simulink model "full_maneuver_single_veh"  (R2020a)
settings: Solver=VariableStepAuto  StartTime=0.0  StopTime=90  FixedStep=0.1  MaxStep=5e-2  RelTol=1e-3
InitFcn:
  | totalVehicles = 5;
  | if exist('vehStatesBus', 'var')==0
  | load vehBuses
  | end
  | if exist('vehErrorsBus', 'var')==0
  | load vehBuses
  | end
libraries: simulink x69, powerlib_meascontrol x6, autolibshared x6, dspsigops x3, eeGeneralControl x2
(part 4 of 6)

== system full_maneuver_single_veh/Fd/Virtual Vehicle Following/Min Velocity Control ==
  ev : Inport
  ea : Inport  Port=2
  realInput : Inport  Port=3
  Abs : Abs
  Compare To Constant : simulink/Logic and Bit Operations/Compare To Constant  relop=<=  const=0.2  OutDataTypeStr=boolean
  Gain : Gain  Gain=velKd
  Scope : Scope  NumInputPorts=4
  Sum1 : Sum  Inputs=|-+
  Sum3 : Sum  Inputs=+++
  Transport Delay : TransportDelay  DelayTime=0.1
  integral term : Subsystem
  velKp : Gain  Gain=velKp
  u : Outport  VectorParamsAs1DForOutWhenUnconnected=off
  wires:
  Gain/1 -> Sum3/3, Scope/3
  ea/1 -> Gain/1
  realInput/1 -> Sum1/1
  Sum3/1 -> u/1, Transport Delay/1, Scope/4
  velKp/1 -> Sum3/2, Scope/2
  ev/1 -> integral term/1(ev), velKp/1
  Sum1/1 -> Abs/1
  Abs/1 -> Compare To Constant/1
  integral term/1(Out1) -> Scope/1, Sum3/1
  Compare To Constant/1 -> integral term/Enable
  Transport Delay/1 -> Sum1/2

== system full_maneuver_single_veh/Fd/Virtual Vehicle Following/Min Velocity Error ==
  ego : Inport
  velRef : Inport  Port=2
  filterReset : Inport  Port=3
  Bus Selector : BusSelector  OutputSignals=Xdot,xddot
  Gain : Gain  Gain=-1
  Gain3 : Gain  Gain=velFilterGain
  Integrator1 : Integrator  ExternalReset=rising  InitialCondition=vx0
  Saturation : Saturate  UpperLimit=maxComfAccel  LowerLimit=minComfAccel
  Sum : Sum  Inputs=+-|
  Sum8 : Sum  Inputs=|+-
  ev : Outport
  ea : Outport  Port=2
  wires:
  Sum8/1 -> Gain3/1
  Gain3/1 -> Saturation/1
  Saturation/1 -> Integrator1/1
  velRef/1 -> Sum8/1
  Integrator1/1 -> Sum/1, Sum8/2
  ego/1 -> Bus Selector/1
  Bus Selector/1 -> Sum/2  "<Xdot>"
  Bus Selector/2 -> Gain/1  "<xddot>"
  Sum/1 -> ev/1
  Gain/1 -> ea/1
  filterReset/1 -> Integrator1/2

== system full_maneuver_single_veh/Fd/Virtual Vehicle Following/Virtual Leader Following ==
  errors : Inport
  errorsDot : Inport  Port=2
  realInput : Inport  Port=3
  leaderChange : Inport  Port=4
  inRange : Inport  Port=5
  Demux : Demux  Outputs=2
  Demux1 : Demux  Outputs=2
  Gain : Gain  Gain=10
  Gain3 : Gain  Gain=Ka
  Gain4 : Gain  Gain=Kdd
  Gain5 : Gain  Gain=10
  Integrator1 : Integrator  ExternalReset=rising  InitialConditionSource=external  InitialCondition=vx0
  Integrator2 : Integrator  ExternalReset=rising
  Kd : Gain  Gain=Kd
  Kp : Gain  Gain=Kp
  Saturation : Saturate  UpperLimit=maxComfAccel  LowerLimit=minAcceleration
  Saturation1 : Saturate  UpperLimit=maxGapError  LowerLimit=-maxGapError*2
  Scope : Scope  NumInputPorts=6
  Sum : Sum  Inputs=+-|
  Sum1 : Sum  Inputs=+++++
  Sum8 : Sum  Inputs=|+-
  Sum9 : Sum  Inputs=|+-
  Transport Delay : TransportDelay  DelayTime=0.1
  integralTerm : Subsystem
  u : Outport  VectorParamsAs1DForOutWhenUnconnected=off
  wires:
  Demux1/2 -> Gain3/1  "evDot"
  Demux1/1 -> Gain4/1  "egDot"
  leaderChange/1 -> integralTerm/3(leaderChange), Integrator2/2
  integralTerm/1(Out1) -> Transport Delay/1
  Sum1/1 -> Sum8/1, Scope/6, Sum/1
  Integrator1/1 -> Sum8/2, u/1
  Gain3/1 -> Sum1/5, Scope/5
  Demux/2 -> Kd/1  "ev"
  Saturation/1 -> Integrator1/1
  Gain4/1 -> Sum1/4, Scope/4
  realInput/1 -> Sum/2, Integrator1/3
  Sum8/1 -> Gain5/1
  Sum/1 -> integralTerm/2(inputDiff)
  Kp/1 -> Sum1/2, Scope/2
  Integrator2/1 -> Sum9/2, Kp/1, integralTerm/1(eh)
  Transport Delay/1 -> Sum1/1, Scope/1
  inRange/1 -> Integrator1/2, integralTerm/Enable
  Gain5/1 -> Saturation/1
  Kd/1 -> Sum1/3, Scope/3
  Demux/1 -> Saturation1/1
  Gain/1 -> Integrator2/1
  Sum9/1 -> Gain/1
  Saturation1/1 -> Sum9/1
  errors/1 -> Demux/1
  errorsDot/1 -> Demux1/1

== system full_maneuver_single_veh/Fd/Virtual Vehicle Following/switch min vel ==
  errors : Inport
  errorsDot : Inport  Port=2
  gap : Inport  Port=3
  h : Inport  Port=4
  d0 : Inport  Port=5
  vRef : Inport  Port=6
  Demux1 : Demux  Outputs=2
  Gain1 : Gain
  MATLAB Function : MATLAB Function  TreatAsAtomicUnit=on
  Relay1 : Relay  OnSwitchValue=1  OffSwitchValue=-1
  Scope : Scope  NumInputPorts=2
  Scope1 : Scope  NumInputPorts=2
  Selector : Selector  InputPortWidth=2  IndexOptions=Index vector (dialog)  Indices=[2]  OutputSizes=1
  Sum2 : Sum  Inputs=-+
  inRange : Outport  VectorParamsAs1DForOutWhenUnconnected=off
  wires:
  d0/1 -> MATLAB Function/2(d0)
  vRef/1 -> MATLAB Function/3(vRef)
  h/1 -> Gain1/1
  errors/1 -> Selector/1
  gap/1 -> Scope/1, Sum2/1
  Sum2/1 -> Scope1/1, Relay1/1
  Selector/1 -> MATLAB Function/4(ev)
  Relay1/1 -> inRange/1, Scope1/2
  Gain1/1 -> MATLAB Function/1(h)
  MATLAB Function/1(maxGap) -> Scope/2, Sum2/2
  errorsDot/1 -> Demux1/1
  Demux1/1 -> MATLAB Function/5(ehDot)
  Demux1/2 -> MATLAB Function/6(ea)

== system full_maneuver_single_veh/Fd_bkp/Find Leader/Subsystem ==
  ego : Inport
  all : Inport  Port=2
  Enable : EnablePort
  MATLAB Function : MATLAB Function  TreatAsAtomicUnit=on
  idx : Outport  InitialOutput=1  VectorParamsAs1DForOutWhenUnconnected=off
  wires:
  all/1 -> MATLAB Function/2(allVehicles)
  MATLAB Function/1(leaderIdx) -> idx/1
  ego/1 -> MATLAB Function/1(ego)

== system full_maneuver_single_veh/Fd_bkp/Find Leader/farAwayVeh ==
  ego : Inport  OutDataTypeStr=Bus: vehStatesBus
  Bus Assignment : BusAssignment  AssignedSignals=X
  Bus Selector : BusSelector  OutputSignals=X
  Constant : Constant  Value=1000
  Sum : Sum  Inputs=|++
  Out1 : Outport  OutDataTypeStr=Bus: vehStatesBus  VectorParamsAs1DForOutWhenUnconnected=off
  wires:
  Sum/1 -> Bus Assignment/2  "X"
  Bus Selector/1 -> Sum/1  "<X>"
  Bus Assignment/1 -> Out1/1
  Constant/1 -> Sum/2
  ego/1 -> Bus Selector/1, Bus Assignment/1

== system full_maneuver_single_veh/Fd_bkp/Lateral Control/Full State Observer ==
  note: xhat
  note: yhat
  measuredOutputs : Inport
  delta : Inport  Port=2
  Add1 : Sum  Inputs=|-+
  Gain : Gain  Gain=B  Multiplication=Matrix(K*u)
  Gain1 : Gain  Gain=C  Multiplication=Matrix(K*u)
  Gain2 : Gain  Gain=L  Multiplication=Matrix(K*u)
  Gain3 : Gain  Gain=A  Multiplication=Matrix(K*u)
  Integrator : Integrator  InitialCondition=[y0; 0; 0; 0]
  Signal Specification : SignalSpecification  Dimensions=[size(C,1) 1]
  Sum : Sum  Inputs=+++
  xhat : Outport  VectorParamsAs1DForOutWhenUnconnected=off
  wires:
  Add1/1 -> Signal Specification/1
  Integrator/1 -> xhat/1, Gain3/1, Gain1/1
  Gain1/1 -> Add1/1
  Sum/1 -> Integrator/1
  measuredOutputs/1 -> Add1/2
  delta/1 -> Gain/1
  Gain/1 -> Sum/3
  Gain3/1 -> Sum/2
  Signal Specification/1 -> Gain2/1
  Gain2/1 -> Sum/1

== system full_maneuver_single_veh/Fd_bkp/Maneuver State/Triggered Subsystem ==
  Trigger : TriggerPort  VariantControl=Variant
  Constant : Constant  OutDataTypeStr=fixdt(1,16,0)
  Out1 : Outport  InitialOutput=0  VectorParamsAs1DForOutWhenUnconnected=off
  wires:
  Constant/1 -> Out1/1

== system full_maneuver_single_veh/Fd_bkp/Maneuver State/Triggered Subsystem1 ==
  Trigger : TriggerPort  VariantControl=Variant
  Constant : Constant  Value=true  OutDataTypeStr=boolean
  Out1 : Outport  OutDataTypeStr=boolean  InitialOutput=0  VectorParamsAs1DForOutWhenUnconnected=off
  wires:
  Constant/1 -> Out1/1

== system full_maneuver_single_veh/Fd_bkp/Maneuver State/safeErrors ==
  errors : Inport
  AND : Logic  Inputs=1  IconShape=distinctive  AllPortsSameDT=off  OutDataTypeStr=boolean
  Compare To Constant4 : simulink/Logic and Bit Operations/Compare To Constant  relop=>=  const=-0.1  OutDataTypeStr=boolean
  Memory : Memory
  Triggered Subsystem1 : Subsystem  TreatAsAtomicUnit=on
  safetyFlag : Outport  VectorParamsAs1DForOutWhenUnconnected=off
  wires:
  Memory/1 -> safetyFlag/1
  Triggered Subsystem1/1(Out1) -> Memory/1
  errors/1 -> Compare To Constant4/1
  AND/1 -> Triggered Subsystem1/Trigger
  Compare To Constant4/1 -> AND/1

== system full_maneuver_single_veh/Fd_bkp/Maneuver State/safeErrors1 ==
  errors : Inport
  AND : Logic  Inputs=1  IconShape=distinctive  AllPortsSameDT=off  OutDataTypeStr=boolean
  Compare To Constant4 : simulink/Logic and Bit Operations/Compare To Constant  relop=>=  const=-0.1  OutDataTypeStr=boolean
  safetyFlag : Outport  VectorParamsAs1DForOutWhenUnconnected=off
  wires:
  AND/1 -> safetyFlag/1
  errors/1 -> Compare To Constant4/1
  Compare To Constant4/1 -> AND/1

== system full_maneuver_single_veh/Fd_bkp/Maneuver State/safeErrors2 ==
  errors : Inport
  AND : Logic  Inputs=1  IconShape=distinctive  AllPortsSameDT=off  OutDataTypeStr=boolean
  Compare To Constant4 : simulink/Logic and Bit Operations/Compare To Constant  relop=>=  const=-0.1  OutDataTypeStr=boolean
  safetyFlag : Outport  VectorParamsAs1DForOutWhenUnconnected=off
  wires:
  errors/1 -> Compare To Constant4/1
  AND/1 -> safetyFlag/1
  Compare To Constant4/1 -> AND/1

== system full_maneuver_single_veh/Fd_bkp/Maneuver State/steadyState ==
  u : Inport
  AND : Logic  Inputs=1  IconShape=distinctive  AllPortsSameDT=off  OutDataTypeStr=boolean
  Abs2 : Abs
  Compare To Constant2 : simulink/Logic and Bit Operations/Compare To Constant  relop=<=  const=0.2  OutDataTypeStr=boolean
  Mux : Mux  Inputs=2
  Transport Delay2 : TransportDelay
  ssFlag : Outport  VectorParamsAs1DForOutWhenUnconnected=off
  wires:
  Mux/1 -> Abs2/1
  AND/1 -> ssFlag/1
  Transport Delay2/1 -> Mux/1
  Abs2/1 -> Compare To Constant2/1
  u/1 -> Mux/2, Transport Delay2/1
  Compare To Constant2/1 -> AND/1

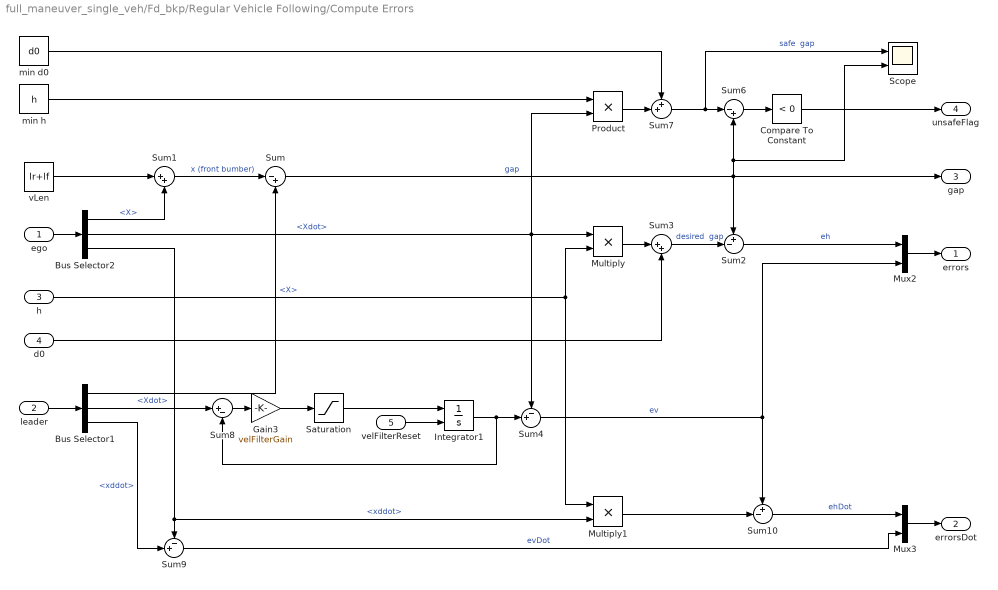
== system full_maneuver_single_veh/Fd_bkp/Regular Vehicle Following/Compute Errors ==
  ego : Inport
  leader : Inport  Port=2
  h : Inport  Port=3
  d0 : Inport  Port=4
  velFilterReset : Inport  Port=5
  Bus Selector1 : BusSelector  OutputSignals=X,Xdot,xddot
  Bus Selector2 : BusSelector  OutputSignals=X,Xdot,xddot
  Compare To Constant : simulink/Logic and Bit Operations/Compare To Constant  relop=<  const=0  OutDataTypeStr=boolean
  Gain3 : Gain  Gain=velFilterGain
  Integrator1 : Integrator  ExternalReset=rising  InitialCondition=vx0
  Multiply : Product
  Multiply1 : Product
  Mux2 : Mux  Inputs=2
  Mux3 : Mux  Inputs=2
  Product : Product
  Saturation : Saturate  UpperLimit=maxAcceleration  LowerLimit=minAcceleration
  Scope : Scope  NumInputPorts=2
  Sum : Sum  Inputs=|-+
  Sum1 : Sum  Inputs=|++
  Sum10 : Sum  Inputs=+-|
  Sum2 : Sum  Inputs=+-|
  Sum3 : Sum  Inputs=|++
  Sum4 : Sum  Inputs=-+|
  Sum6 : Sum  Inputs=|-+
  Sum7 : Sum  Inputs=++|
  Sum8 : Sum  Inputs=|+-
  Sum9 : Sum  Inputs=-+|
  min d0 : Constant  Value=d0
  min h : Constant  Value=h
  vLen : Constant  Value=lr+lf
  errors : Outport  VectorParamsAs1DForOutWhenUnconnected=off
  errorsDot : Outport  Port=2
  "gap " : Outport  Port=3  VectorParamsAs1DForOutWhenUnconnected=off
  unsafeFlag : Outport  Port=4  VectorParamsAs1DForOutWhenUnconnected=off
  wires:
  Mux2/1 -> errors/1
  velFilterReset/1 -> Integrator1/2
  Sum6/1 -> Compare To Constant/1
  Sum7/1 -> Sum6/1, Scope/1  "safe  gap"
  min h/1 -> Product/1
  Compare To Constant/1 -> unsafeFlag/1
  Sum2/1 -> Mux2/1  "eh"
  Bus Selector1/1 -> Sum/2  "<X>"
  Product/1 -> Sum7/2
  Sum3/1 -> Sum2/2  "desired  gap"
  Sum1/1 -> Sum/1  "x (front bumber)"
  Bus Selector2/2 -> Sum4/1, Multiply/1, Product/2  "<Xdot>"
  d0/1 -> Sum3/2
  vLen/1 -> Sum1/1
  min d0/1 -> Sum7/1
  Multiply/1 -> Sum3/1
  Sum/1 -> Sum2/1, "gap "/1, Sum6/2, Scope/2  "gap"
  Bus Selector2/1 -> Sum1/2  "<X>"
  h/1 -> Multiply/2, Multiply1/1
  Bus Selector1/2 -> Sum8/1  "<Xdot>"
  Sum4/1 -> Mux2/2, Sum10/1  "ev"
  Gain3/1 -> Saturation/1
  Saturation/1 -> Integrator1/1
  Integrator1/1 -> Sum4/2, Sum8/2
  Sum8/1 -> Gain3/1
  Bus Selector1/3 -> Sum9/2  "<xddot>"
  Bus Selector2/3 -> Sum9/1, Multiply1/2  "<xddot>"
  Multiply1/1 -> Sum10/2
  Sum10/1 -> Mux3/1  "ehDot"
  Sum9/1 -> Mux3/2  "evDot"
  Mux3/1 -> errorsDot/1
  ego/1 -> Bus Selector2/1
  leader/1 -> Bus Selector1/1

== system full_maneuver_single_veh/Fd_bkp/Regular Vehicle Following/Define Desired Distance ==
  extraSpaceFlag : Inport
  Constant : Constant  Value=h
  Constant1 : Constant  Value=d0
  Constant2 : Constant  Value=hLC
  Constant3 : Constant  Value=d0LC
  Demux : Demux  Outputs=2
  Integrator : Integrator  InitialCondition=[h d0]
  Mux : Mux  Inputs=2
  Mux1 : Mux  Inputs=2
  Saturation1 : Saturate  UpperLimit=hFilterSaturation  LowerLimit=-hFilterSaturation
  Sum5 : Sum  Inputs=|+-
  Switch : Switch  Criteria=u2 > Threshold
  hFilterGain : Gain  Gain=hFilterGain
  h : Outport
  d0 : Outport  Port=2
  wires:
  Mux/1 -> Switch/3
  Constant/1 -> Mux/1
  hFilterGain/1 -> Saturation1/1
  Constant2/1 -> Mux1/1
  Sum5/1 -> hFilterGain/1
  Mux1/1 -> Switch/1
  Switch/1 -> Sum5/1
  Constant3/1 -> Mux1/2
  Constant1/1 -> Mux/2
  extraSpaceFlag/1 -> Switch/2
  Saturation1/1 -> Integrator/1
  Integrator/1 -> Demux/1, Sum5/2
  Demux/1 -> h/1
  Demux/2 -> d0/1

== system full_maneuver_single_veh/Fd_bkp/Regular Vehicle Following/Veh Following ==
  errors : Inport
  errorsDot : Inport  Port=2
  realInput : Inport  Port=3
  leaderChange : Inport  Port=4
  inRange : Inport  Port=5
  Demux : Demux  Outputs=2
  Demux1 : Demux  Outputs=2
  Gain : Gain  Gain=Ka
  Gain1 : Gain  Gain=Kdd
  Kd : Gain  Gain=Kd
  Kp : Gain  Gain=Kp
  Saturation1 : Saturate  UpperLimit=maxHeadwayError  LowerLimit=minHeadwayError
  Scope : Scope  NumInputPorts=6
  Sum : Sum  Inputs=|-+
  Sum1 : Sum  Inputs=+++
  Sum2 : Sum  Inputs=|++
  Sum3 : Sum  Inputs=|++
  Transport Delay : TransportDelay  DelayTime=0.1
  integralTerm : Subsystem
  u : Outport  VectorParamsAs1DForOutWhenUnconnected=off
  wires:
  inRange/1 -> integralTerm/Enable
  errors/1 -> Demux/1
  Saturation1/1 -> integralTerm/1(eh), Kp/1
  Demux/2 -> Kd/1  "ev"
  Kp/1 -> Sum1/2, Scope/2
  Kd/1 -> Scope/3, Sum1/3
  Demux/1 -> Saturation1/1  "eh"
  leaderChange/1 -> integralTerm/2(leaderChange)
  Transport Delay/1 -> Sum1/1, Scope/1
  Sum1/1 -> Sum3/1
  realInput/1 -> Sum/1
  Sum/1 -> integralTerm/3(inputDiff)
  integralTerm/1(Out1) -> Transport Delay/1
  Gain1/1 -> Scope/4, Sum2/1
  Gain/1 -> Scope/5, Sum2/2
  Sum3/1 -> Scope/6, Sum/2, u/1
  Sum2/1 -> Sum3/2
  errorsDot/1 -> Demux1/1
  Demux1/1 -> Gain1/1  "ehDot"
  Demux1/2 -> Gain/1  "evDot"

== system full_maneuver_single_veh/Fd_bkp/Regular Vehicle Following/Velocity Control ==
  ev : Inport
  ea : Inport  Port=2
  realInput : Inport  Port=3
  Abs : Abs
  Compare To Constant : simulink/Logic and Bit Operations/Compare To Constant  relop=<=  const=0.5  OutDataTypeStr=boolean
  Gain : Gain  Gain=velKd
  Scope : Scope  NumInputPorts=4
  Sum1 : Sum  Inputs=|-+
  Sum3 : Sum  Inputs=+++
  Transport Delay : TransportDelay  DelayTime=0.1
  integral term : Subsystem
  velKp : Gain  Gain=velKp
  u : Outport  VectorParamsAs1DForOutWhenUnconnected=off
  wires:
  Gain/1 -> Sum3/3, Scope/3
  ea/1 -> Gain/1
  realInput/1 -> Sum1/1
  Sum3/1 -> u/1, Transport Delay/1, Scope/4
  velKp/1 -> Sum3/2, Scope/2
  ev/1 -> integral term/1(ev), velKp/1
  Sum1/1 -> Abs/1
  Abs/1 -> Compare To Constant/1
  integral term/1(Out1) -> Scope/1, Sum3/1
  Compare To Constant/1 -> integral term/Enable
  Transport Delay/1 -> Sum1/2

== system full_maneuver_single_veh/Fd_bkp/Regular Vehicle Following/switch free flow ==
  errors : Inport
  errorsDot : Inport  Port=2
  gap : Inport  Port=3
  h : Inport  Port=4
  d0 : Inport  Port=5
  vRef : Inport  Port=6
  Demux1 : Demux  Outputs=2
  Gain1 : Gain
  MATLAB Function : MATLAB Function  TreatAsAtomicUnit=on
  Relay : Relay  OnSwitchValue=1  OffSwitchValue=-1
  Scope : Scope  NumInputPorts=2
  Selector : Selector  InputPortWidth=2  IndexOptions=Index vector (dialog)  Indices=[2]  OutputSizes=1
  Sum2 : Sum  Inputs=-+
  inRange : Outport  VectorParamsAs1DForOutWhenUnconnected=off
  wires:
  d0/1 -> MATLAB Function/2(d0)
  vRef/1 -> MATLAB Function/3(vRef)
  h/1 -> Gain1/1
  errors/1 -> Selector/1
  gap/1 -> Scope/1, Sum2/1
  Sum2/1 -> Relay/1
  Selector/1 -> MATLAB Function/4(ev)
  Relay/1 -> inRange/1
  Gain1/1 -> MATLAB Function/1(h)
  MATLAB Function/1(maxGap) -> Scope/2, Sum2/2
  errorsDot/1 -> Demux1/1
  Demux1/1 -> MATLAB Function/5(ehDot)
  Demux1/2 -> MATLAB Function/6(ea)

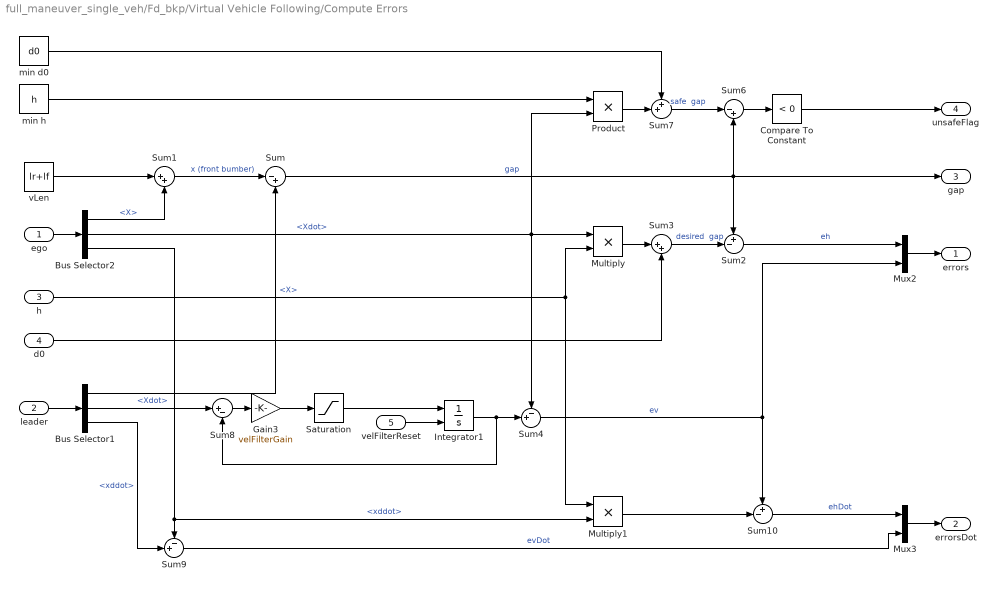
== system full_maneuver_single_veh/Fd_bkp/Virtual Vehicle Following/Compute Errors ==
  ego : Inport
  leader : Inport  Port=2
  h : Inport  Port=3
  d0 : Inport  Port=4
  velFilterReset : Inport  Port=5
  Bus Selector1 : BusSelector  OutputSignals=X,Xdot,xddot
  Bus Selector2 : BusSelector  OutputSignals=X,Xdot,xddot
  Compare To Constant : simulink/Logic and Bit Operations/Compare To Constant  relop=<  const=0  OutDataTypeStr=boolean
  Gain3 : Gain  Gain=velFilterGain
  Integrator1 : Integrator  ExternalReset=rising  InitialCondition=vx0
  Multiply : Product
  Multiply1 : Product
  Mux2 : Mux  Inputs=2
  Mux3 : Mux  Inputs=2
  Product : Product
  Saturation : Saturate  UpperLimit=maxAcceleration  LowerLimit=minAcceleration
  Sum : Sum  Inputs=|-+
  Sum1 : Sum  Inputs=|++
  Sum10 : Sum  Inputs=+-|
  Sum2 : Sum  Inputs=+-|
  Sum3 : Sum  Inputs=|++
  Sum4 : Sum  Inputs=-+|
  Sum6 : Sum  Inputs=|-+
  Sum7 : Sum  Inputs=++|
  Sum8 : Sum  Inputs=|+-
  Sum9 : Sum  Inputs=-+|
  min d0 : Constant  Value=d0
  min h : Constant  Value=h
  vLen : Constant  Value=lr+lf
  errors : Outport  VectorParamsAs1DForOutWhenUnconnected=off
  errorsDot : Outport  Port=2
  "gap " : Outport  Port=3  VectorParamsAs1DForOutWhenUnconnected=off
  unsafeFlag : Outport  Port=4  VectorParamsAs1DForOutWhenUnconnected=off
  wires:
  Mux2/1 -> errors/1
  velFilterReset/1 -> Integrator1/2
  Sum6/1 -> Compare To Constant/1
  Sum7/1 -> Sum6/1  "safe  gap"
  min h/1 -> Product/1
  Compare To Constant/1 -> unsafeFlag/1
  Sum2/1 -> Mux2/1  "eh"
  Bus Selector1/1 -> Sum/2  "<X>"
  Product/1 -> Sum7/2
  Sum3/1 -> Sum2/2  "desired  gap"
  Sum1/1 -> Sum/1  "x (front bumber)"
  Bus Selector2/2 -> Sum4/1, Multiply/1, Product/2  "<Xdot>"
  d0/1 -> Sum3/2
  vLen/1 -> Sum1/1
  min d0/1 -> Sum7/1
  Multiply/1 -> Sum3/1
  Sum/1 -> Sum2/1, "gap "/1, Sum6/2  "gap"
  Bus Selector2/1 -> Sum1/2  "<X>"
  h/1 -> Multiply/2, Multiply1/1
  Bus Selector1/2 -> Sum8/1  "<Xdot>"
  Sum4/1 -> Mux2/2, Sum10/1  "ev"
  Gain3/1 -> Saturation/1
  Saturation/1 -> Integrator1/1
  Integrator1/1 -> Sum4/2, Sum8/2
  Sum8/1 -> Gain3/1
  Bus Selector1/3 -> Sum9/2  "<xddot>"
  Bus Selector2/3 -> Sum9/1, Multiply1/2  "<xddot>"
  Multiply1/1 -> Sum10/2
  Sum10/1 -> Mux3/1  "ehDot"
  Sum9/1 -> Mux3/2  "evDot"
  Mux3/1 -> errorsDot/1
  ego/1 -> Bus Selector2/1
  leader/1 -> Bus Selector1/1

== system full_maneuver_single_veh/Fd_bkp/Virtual Vehicle Following/Define Desired Distance ==
  extraSpaceFlag : Inport
  Constant : Constant  Value=h
  Constant1 : Constant  Value=d0
  Constant2 : Constant  Value=hLC
  Constant3 : Constant  Value=d0LC
  Demux : Demux  Outputs=2
  Integrator : Integrator  InitialCondition=[h d0]
  Mux : Mux  Inputs=2
  Mux1 : Mux  Inputs=2
  Saturation1 : Saturate  UpperLimit=hFilterSaturation  LowerLimit=-hFilterSaturation
  Sum5 : Sum  Inputs=|+-
  Switch : Switch  Criteria=u2 > Threshold
  hFilterGain : Gain  Gain=hFilterGain
  h : Outport
  d0 : Outport  Port=2
  wires:
  Mux/1 -> Switch/3
  Constant/1 -> Mux/1
  hFilterGain/1 -> Saturation1/1
  Constant2/1 -> Mux1/1
  Sum5/1 -> hFilterGain/1
  Mux1/1 -> Switch/1
  Switch/1 -> Sum5/1
  Constant3/1 -> Mux1/2
  Constant1/1 -> Mux/2
  extraSpaceFlag/1 -> Switch/2
  Saturation1/1 -> Integrator/1
  Integrator/1 -> Demux/1, Sum5/2
  Demux/1 -> h/1
  Demux/2 -> d0/1

== system full_maneuver_single_veh/Fd_bkp/Virtual Vehicle Following/Velocity Control1 ==
  ev : Inport
  ea : Inport  Port=2
  realInput : Inport  Port=3
  Abs : Abs
  Compare To Constant : simulink/Logic and Bit Operations/Compare To Constant  relop=<=  const=0.5  OutDataTypeStr=boolean
  Gain : Gain  Gain=velKd
  Scope : Scope  NumInputPorts=4
  Sum1 : Sum  Inputs=|-+
  Sum3 : Sum  Inputs=+++
  Transport Delay : TransportDelay  DelayTime=0.1
  integral term : Subsystem
  velKp : Gain  Gain=velKp
  u : Outport  VectorParamsAs1DForOutWhenUnconnected=off
  wires:
  Gain/1 -> Sum3/3, Scope/3
  ea/1 -> Gain/1
  realInput/1 -> Sum1/1
  Sum3/1 -> u/1, Transport Delay/1, Scope/4
  velKp/1 -> Sum3/2, Scope/2
  ev/1 -> integral term/1(ev), velKp/1
  Sum1/1 -> Abs/1
  Abs/1 -> Compare To Constant/1
  integral term/1(Out1) -> Scope/1, Sum3/1
  Compare To Constant/1 -> integral term/Enable
  Transport Delay/1 -> Sum1/2

== system full_maneuver_single_veh/Fd_bkp/Virtual Vehicle Following/Velocity Control2 ==
  ev : Inport
  ea : Inport  Port=2
  realInput : Inport  Port=3
  Abs : Abs
  Compare To Constant : simulink/Logic and Bit Operations/Compare To Constant  relop=<=  const=0.5  OutDataTypeStr=boolean
  Gain : Gain  Gain=velKd
  Scope : Scope  NumInputPorts=4
  Sum1 : Sum  Inputs=|-+
  Sum3 : Sum  Inputs=+++
  Transport Delay : TransportDelay  DelayTime=0.1
  integral term : Subsystem
  velKp : Gain  Gain=velKp
  u : Outport  VectorParamsAs1DForOutWhenUnconnected=off
  wires:
  Transport Delay/1 -> Sum1/2
  Compare To Constant/1 -> integral term/Enable
  integral term/1(Out1) -> Sum3/1, Scope/1
  Abs/1 -> Compare To Constant/1
  Sum1/1 -> Abs/1
  ev/1 -> velKp/1, integral term/1(ev)
  velKp/1 -> Scope/2, Sum3/2
  Sum3/1 -> Scope/4, Transport Delay/1, u/1
  realInput/1 -> Sum1/1
  ea/1 -> Gain/1
  Gain/1 -> Scope/3, Sum3/3

== system full_maneuver_single_veh/Fd_bkp/Virtual Vehicle Following/Virtual Leader Following ==
  errors : Inport
  errorsDot : Inport  Port=2
  realInput : Inport  Port=3
  leaderChange : Inport  Port=4
  inRange : Inport  Port=5
  Demux : Demux  Outputs=2
  Demux1 : Demux  Outputs=2
  Gain : Gain  Gain=10
  Gain1 : Gain  Gain=Ka
  Gain2 : Gain  Gain=Kdd
  Integrator2 : Integrator  ExternalReset=rising
  Kd : Gain  Gain=Kd
  Kp : Gain  Gain=Kp
  Saturation1 : Saturate  UpperLimit=maxHeadwayError  LowerLimit=-maxHeadwayError*2
  Scope1 : Scope  NumInputPorts=6
  Sum : Sum  Inputs=|-+
  Sum1 : Sum  Inputs=+++
  Sum2 : Sum  Inputs=|++
  Sum3 : Sum  Inputs=|++
  Sum9 : Sum  Inputs=|+-
  Transport Delay : TransportDelay  DelayTime=0.1
  integralTerm : Subsystem
  u : Outport  VectorParamsAs1DForOutWhenUnconnected=off
  wires:
  leaderChange/1 -> Integrator2/2, integralTerm/2(leaderChange)
  Demux/1 -> Saturation1/1
  Integrator2/1 -> Kp/1, integralTerm/1(eh), Sum9/2
  Kd/1 -> Sum1/3, Scope1/3
  Kp/1 -> Sum1/2, Scope1/2
  Demux/2 -> Kd/1
  Gain/1 -> Integrator2/1
  Sum9/1 -> Gain/1
  Saturation1/1 -> Sum9/1
  integralTerm/1(Out1) -> Transport Delay/1
  inRange/1 -> integralTerm/Enable
  errors/1 -> Demux/1
  realInput/1 -> Sum/1
  Sum1/1 -> Sum3/1
  Sum/1 -> integralTerm/3(inputDiff)
  Transport Delay/1 -> Sum1/1, Scope1/1
  Sum3/1 -> Sum/2, u/1, Scope1/6
  Gain1/1 -> Sum2/2, Scope1/5
  Gain2/1 -> Sum2/1, Scope1/4
  Demux1/2 -> Gain1/1  "evDot"
  Sum2/1 -> Sum3/2
  errorsDot/1 -> Demux1/1
  Demux1/1 -> Gain2/1  "ehDot"

== system full_maneuver_single_veh/Fd_bkp/Virtual Vehicle Following/switch free flow ==
  errors : Inport
  errorsDot : Inport  Port=2
  gap : Inport  Port=3
  h : Inport  Port=4
  d0 : Inport  Port=5
  vRef : Inport  Port=6
  Demux1 : Demux  Outputs=2
  Gain1 : Gain
  MATLAB Function : MATLAB Function  TreatAsAtomicUnit=on
  Relay : Relay  OnSwitchValue=1  OffSwitchValue=-1
  Scope : Scope  NumInputPorts=2
  Selector : Selector  InputPortWidth=2  IndexOptions=Index vector (dialog)  Indices=[2]  OutputSizes=1
  Sum2 : Sum  Inputs=-+
  inRange : Outport  VectorParamsAs1DForOutWhenUnconnected=off
  wires:
  d0/1 -> MATLAB Function/2(d0)
  vRef/1 -> MATLAB Function/3(vRef)
  h/1 -> Gain1/1
  errors/1 -> Selector/1
  gap/1 -> Scope/1, Sum2/1
  Sum2/1 -> Relay/1
  Selector/1 -> MATLAB Function/4(ev)
  Relay/1 -> inRange/1
  Gain1/1 -> MATLAB Function/1(h)
  MATLAB Function/1(maxGap) -> Scope/2, Sum2/2
  errorsDot/1 -> Demux1/1
  Demux1/1 -> MATLAB Function/5(ehDot)
  Demux1/2 -> MATLAB Function/6(ea)

== system full_maneuver_single_veh/Fd_bkp/Virtual Vehicle Following/switch min vel ==
  errors : Inport
  errorsDot : Inport  Port=2
  gap : Inport  Port=3
  h : Inport  Port=4
  d0 : Inport  Port=5
  vRef : Inport  Port=6
  Demux1 : Demux  Outputs=2
  Gain1 : Gain
  MATLAB Function : MATLAB Function  TreatAsAtomicUnit=on
  Relay1 : Relay  OnSwitchValue=1  OffSwitchValue=-1
  Scope : Scope  NumInputPorts=2
  Scope1 : Scope  NumInputPorts=2
  Selector : Selector  InputPortWidth=2  IndexOptions=Index vector (dialog)  Indices=[2]  OutputSizes=1
  Sum2 : Sum  Inputs=-+
  inRange : Outport  VectorParamsAs1DForOutWhenUnconnected=off
  wires:
  d0/1 -> MATLAB Function/2(d0)
  vRef/1 -> MATLAB Function/3(vRef)
  h/1 -> Gain1/1
  errors/1 -> Selector/1
  gap/1 -> Scope/1, Sum2/1
  Sum2/1 -> Scope1/1, Relay1/1
  Selector/1 -> MATLAB Function/4(ev)
  Relay1/1 -> inRange/1, Scope1/2
  Gain1/1 -> MATLAB Function/1(h)
  MATLAB Function/1(maxGap) -> Scope/2, Sum2/2
  errorsDot/1 -> Demux1/1
  Demux1/1 -> MATLAB Function/5(ehDot)
  Demux1/2 -> MATLAB Function/6(ea)

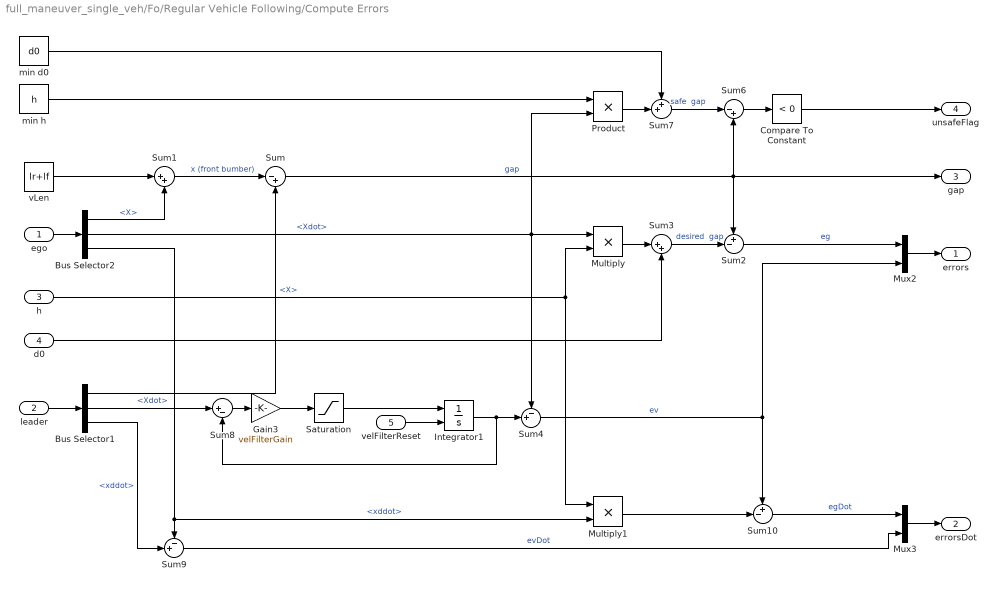
== system full_maneuver_single_veh/Fo/Regular Vehicle Following/Compute Errors ==
  ego : Inport
  leader : Inport  Port=2
  h : Inport  Port=3
  d0 : Inport  Port=4
  velFilterReset : Inport  Port=5
  Bus Selector1 : BusSelector  OutputSignals=X,Xdot,xddot
  Bus Selector2 : BusSelector  OutputSignals=X,Xdot,xddot
  Compare To Constant : simulink/Logic and Bit Operations/Compare To Constant  relop=<  const=0  OutDataTypeStr=boolean
  Gain3 : Gain  Gain=velFilterGain
  Integrator1 : Integrator  ExternalReset=rising  InitialCondition=vx0
  Multiply : Product
  Multiply1 : Product
  Mux2 : Mux  Inputs=2
  Mux3 : Mux  Inputs=2
  Product : Product
  Saturation : Saturate  UpperLimit=maxAcceleration  LowerLimit=minAcceleration
  Sum : Sum  Inputs=|-+
  Sum1 : Sum  Inputs=|++
  Sum10 : Sum  Inputs=+-|
  Sum2 : Sum  Inputs=+-|
  Sum3 : Sum  Inputs=|++
  Sum4 : Sum  Inputs=-+|
  Sum6 : Sum  Inputs=|-+
  Sum7 : Sum  Inputs=++|
  Sum8 : Sum  Inputs=|+-
  Sum9 : Sum  Inputs=-+|
  min d0 : Constant  Value=d0
  min h : Constant  Value=h
  vLen : Constant  Value=lr+lf
  errors : Outport  VectorParamsAs1DForOutWhenUnconnected=off
  errorsDot : Outport  Port=2
  "gap " : Outport  Port=3  VectorParamsAs1DForOutWhenUnconnected=off
  unsafeFlag : Outport  Port=4  VectorParamsAs1DForOutWhenUnconnected=off
  wires:
  Mux2/1 -> errors/1
  velFilterReset/1 -> Integrator1/2
  Sum6/1 -> Compare To Constant/1
  Sum7/1 -> Sum6/1  "safe  gap"
  min h/1 -> Product/1
  Compare To Constant/1 -> unsafeFlag/1
  Sum2/1 -> Mux2/1  "eg"
  Bus Selector1/1 -> Sum/2  "<X>"
  Product/1 -> Sum7/2
  Sum3/1 -> Sum2/2  "desired  gap"
  Sum1/1 -> Sum/1  "x (front bumber)"
  Bus Selector2/2 -> Sum4/1, Multiply/1, Product/2  "<Xdot>"
  d0/1 -> Sum3/2
  vLen/1 -> Sum1/1
  min d0/1 -> Sum7/1
  Multiply/1 -> Sum3/1
  Sum/1 -> Sum2/1, "gap "/1, Sum6/2  "gap"
  Bus Selector2/1 -> Sum1/2  "<X>"
  h/1 -> Multiply/2, Multiply1/1
  Bus Selector1/2 -> Sum8/1  "<Xdot>"
  Sum4/1 -> Mux2/2, Sum10/1  "ev"
  Gain3/1 -> Saturation/1
  Saturation/1 -> Integrator1/1
  Integrator1/1 -> Sum4/2, Sum8/2
  Sum8/1 -> Gain3/1
  Bus Selector1/3 -> Sum9/2  "<xddot>"
  Bus Selector2/3 -> Sum9/1, Multiply1/2  "<xddot>"
  Multiply1/1 -> Sum10/2
  Sum10/1 -> Mux3/1  "egDot"
  Sum9/1 -> Mux3/2  "evDot"
  Mux3/1 -> errorsDot/1
  ego/1 -> Bus Selector2/1
  leader/1 -> Bus Selector1/1

== system full_maneuver_single_veh/Fo/Regular Vehicle Following/Define Desired Distance ==
  extraSpaceFlag : Inport
  Constant : Constant  Value=h
  Constant1 : Constant  Value=d0
  Constant2 : Constant  Value=hLC
  Constant3 : Constant  Value=d0LC
  Demux : Demux  Outputs=2
  Integrator : Integrator  InitialCondition=[h d0]
  Mux : Mux  Inputs=2
  Mux1 : Mux  Inputs=2
  Saturation1 : Saturate  UpperLimit=hFilterSaturation  LowerLimit=-hFilterSaturation
  Sum5 : Sum  Inputs=|+-
  Switch : Switch  Criteria=u2 > Threshold
  hFilterGain : Gain  Gain=hFilterGain
  h : Outport
  d0 : Outport  Port=2
  wires:
  Mux/1 -> Switch/3
  Constant/1 -> Mux/1
  hFilterGain/1 -> Saturation1/1
  Constant2/1 -> Mux1/1
  Sum5/1 -> hFilterGain/1
  Mux1/1 -> Switch/1
  Switch/1 -> Sum5/1
  Constant3/1 -> Mux1/2
  Constant1/1 -> Mux/2
  extraSpaceFlag/1 -> Switch/2
  Saturation1/1 -> Integrator/1
  Integrator/1 -> Demux/1, Sum5/2
  Demux/1 -> h/1
  Demux/2 -> d0/1

== system full_maneuver_single_veh/Fo/Regular Vehicle Following/Veh Following ==
  errors : Inport
  errorsDot : Inport  Port=2
  realInput : Inport  Port=3
  leaderChange : Inport  Port=4
  inRange : Inport  Port=5
  Demux : Demux  Outputs=2
  Demux1 : Demux  Outputs=2
  Gain : Gain  Gain=Ka
  Gain1 : Gain  Gain=Kdd
  Gain3 : Gain  Gain=10
  Integrator1 : Integrator  ExternalReset=rising  InitialConditionSource=external  InitialCondition=vx0
  Kd : Gain  Gain=Kd
  Kp : Gain  Gain=Kp
  Saturation : Saturate  UpperLimit=inf  LowerLimit=minAcceleration
  Saturation1 : Saturate  UpperLimit=maxGapError  LowerLimit=minGapError
  Scope : Scope  NumInputPorts=6
  Sum : Sum  Inputs=+-|
  Sum1 : Sum  Inputs=+++++
  Sum8 : Sum  Inputs=|+-
  Transport Delay : TransportDelay  DelayTime=0.1
  integralTerm : Subsystem
  u : Outport  VectorParamsAs1DForOutWhenUnconnected=off
  wires:
  Kp/1 -> Sum1/2, Scope/2
  Gain3/1 -> Saturation/1
  Sum8/1 -> Gain3/1
  Saturation/1 -> Integrator1/1
  Integrator1/1 -> u/1, Sum8/2
  errors/1 -> Demux/1
  Saturation1/1 -> integralTerm/1(eh), Kp/1
  Demux/2 -> Kd/1  "ev"
  Kd/1 -> Sum1/3, Scope/3
  Demux/1 -> Saturation1/1  "eg"
  leaderChange/1 -> integralTerm/3(leaderChange)
  inRange/1 -> Integrator1/2, integralTerm/Enable
  Transport Delay/1 -> Sum1/1, Scope/1
  realInput/1 -> Sum/2, Integrator1/3
  Sum/1 -> integralTerm/2(inputDiff)
  integralTerm/1(Out1) -> Transport Delay/1
  Gain1/1 -> Sum1/4, Scope/4
  Gain/1 -> Sum1/5, Scope/5
  Sum1/1 -> Sum8/1, Sum/1, Scope/6
  errorsDot/1 -> Demux1/1
  Demux1/1 -> Gain1/1  "egDot"
  Demux1/2 -> Gain/1  "evDot"

== system full_maneuver_single_veh/Fo/Regular Vehicle Following/Velocity Control ==
  ev : Inport
  ea : Inport  Port=2
  realInput : Inport  Port=3
  Abs : Abs
  Compare To Constant : simulink/Logic and Bit Operations/Compare To Constant  relop=<=  const=0.5  OutDataTypeStr=boolean
  Constant : Constant  Value=0.05
  Gain : Gain  Gain=velKd
  Scope : Scope  NumInputPorts=4
  Sum : Sum  Inputs=++|
  Sum1 : Sum  Inputs=|-+
  Sum3 : Sum  Inputs=+++
  Transport Delay : TransportDelay  DelayTime=0.1
  integral term : Subsystem
  velKp : Gain  Gain=velKp
  u : Outport  VectorParamsAs1DForOutWhenUnconnected=off
  wires:
  Sum/1 -> u/1
  Constant/1 -> Sum/1
  Gain/1 -> Sum3/3, Scope/3
  ea/1 -> Gain/1
  realInput/1 -> Sum1/1
  Sum3/1 -> Transport Delay/1, Scope/4, Sum/2
  velKp/1 -> Sum3/2, Scope/2
  ev/1 -> integral term/1(ev), velKp/1
  Sum1/1 -> Abs/1
  Abs/1 -> Compare To Constant/1
  integral term/1(Out1) -> Scope/1, Sum3/1
  Compare To Constant/1 -> integral term/Enable
  Transport Delay/1 -> Sum1/2

== system full_maneuver_single_veh/Fo/Regular Vehicle Following/Velocity Error ==
  ego : Inport
  velRef : Inport  Port=2
  inRange : Inport  Port=3
  Bus Selector : BusSelector  OutputSignals=Xdot,xddot
  Gain : Gain  Gain=-1
  Gain3 : Gain  Gain=velFilterGain
  Integrator1 : Integrator  ExternalReset=rising  InitialCondition=vx0
  Saturation : Saturate  UpperLimit=maxComfAccel  LowerLimit=minComfAccel
  Sum : Sum  Inputs=+-|
  Sum8 : Sum  Inputs=|+-
  ev : Outport
  ea : Outport  Port=2
  wires:
  inRange/1 -> Integrator1/2
  Gain/1 -> ea/1
  Sum/1 -> ev/1
  Bus Selector/2 -> Gain/1  "<xddot>"
  Bus Selector/1 -> Sum/2  "<Xdot>"
  ego/1 -> Bus Selector/1
  Integrator1/1 -> Sum8/2, Sum/1
  velRef/1 -> Sum8/1
  Saturation/1 -> Integrator1/1
  Gain3/1 -> Saturation/1
  Sum8/1 -> Gain3/1

== system full_maneuver_single_veh/Fo/Regular Vehicle Following/switch ==
  errors : Inport
  errorsDot : Inport  Port=2
  gap : Inport  Port=3
  h : Inport  Port=4
  d0 : Inport  Port=5
  vRef : Inport  Port=6
  Compare To Constant : simulink/Logic and Bit Operations/Compare To Constant  relop=<=  const=0  OutDataTypeStr=boolean
  Demux1 : Demux  Outputs=2
  Gain1 : Gain
  MATLAB Function : MATLAB Function  TreatAsAtomicUnit=on
  Scope : Scope  NumInputPorts=2
  Selector : Selector  InputPortWidth=2  IndexOptions=Index vector (dialog)  Indices=[2]  OutputSizes=1
  Sum2 : Sum  Inputs=+-
  inRange : Outport  VectorParamsAs1DForOutWhenUnconnected=off
  wires:
  d0/1 -> MATLAB Function/2(d0)
  vRef/1 -> MATLAB Function/3(vRef)
  h/1 -> Gain1/1
  errors/1 -> Selector/1
  gap/1 -> Scope/1, Sum2/1
  Sum2/1 -> Compare To Constant/1
  Selector/1 -> MATLAB Function/4(ev)
  Compare To Constant/1 -> inRange/1
  Gain1/1 -> MATLAB Function/1(h)
  MATLAB Function/1(maxGap) -> Scope/2, Sum2/2
  errorsDot/1 -> Demux1/1
  Demux1/1 -> MATLAB Function/5(ehDot)
  Demux1/2 -> MATLAB Function/6(ea)

== system full_maneuver_single_veh/Fo/findLeader/Subsystem ==
  ego : Inport
  all : Inport  Port=2
  Enable : EnablePort
  MATLAB Function : MATLAB Function  TreatAsAtomicUnit=on
  idx : Outport  InitialOutput=1  VectorParamsAs1DForOutWhenUnconnected=off
  wires:
  all/1 -> MATLAB Function/2(allVehicles)
  MATLAB Function/1(leaderIdx) -> idx/1
  ego/1 -> MATLAB Function/1(ego)

== system full_maneuver_single_veh/Fo/findLeader/farAwayVeh ==
  ego : Inport  OutDataTypeStr=Bus: vehStatesBus
  Bus Assignment : BusAssignment  AssignedSignals=X
  Bus Selector : BusSelector  OutputSignals=X
  Constant : Constant  Value=1000
  Sum : Sum  Inputs=|++
  Out1 : Outport  OutDataTypeStr=Bus: vehStatesBus  VectorParamsAs1DForOutWhenUnconnected=off
  wires:
  ego/1 -> Bus Assignment/1, Bus Selector/1
  Constant/1 -> Sum/2
  Bus Assignment/1 -> Out1/1
  Bus Selector/1 -> Sum/1  "<X>"
  Sum/1 -> Bus Assignment/2  "X"

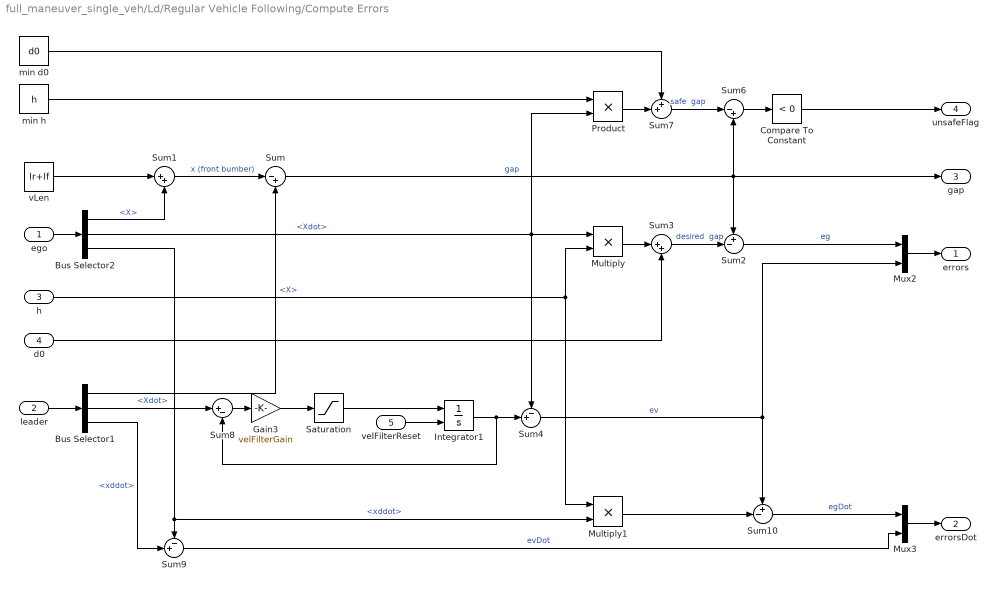
== system full_maneuver_single_veh/Ld/Regular Vehicle Following/Compute Errors ==
  ego : Inport
  leader : Inport  Port=2
  h : Inport  Port=3
  d0 : Inport  Port=4
  velFilterReset : Inport  Port=5
  Bus Selector1 : BusSelector  OutputSignals=X,Xdot,xddot
  Bus Selector2 : BusSelector  OutputSignals=X,Xdot,xddot
  Compare To Constant : simulink/Logic and Bit Operations/Compare To Constant  relop=<  const=0  OutDataTypeStr=boolean
  Gain3 : Gain  Gain=velFilterGain
  Integrator1 : Integrator  ExternalReset=rising  InitialCondition=vx0
  Multiply : Product
  Multiply1 : Product
  Mux2 : Mux  Inputs=2
  Mux3 : Mux  Inputs=2
  Product : Product
  Saturation : Saturate  UpperLimit=maxAcceleration  LowerLimit=minAcceleration
  Sum : Sum  Inputs=|-+
  Sum1 : Sum  Inputs=|++
  Sum10 : Sum  Inputs=+-|
  Sum2 : Sum  Inputs=+-|
  Sum3 : Sum  Inputs=|++
  Sum4 : Sum  Inputs=-+|
  Sum6 : Sum  Inputs=|-+
  Sum7 : Sum  Inputs=++|
  Sum8 : Sum  Inputs=|+-
  Sum9 : Sum  Inputs=-+|
  min d0 : Constant  Value=d0
  min h : Constant  Value=h
  vLen : Constant  Value=lr+lf
  errors : Outport  VectorParamsAs1DForOutWhenUnconnected=off
  errorsDot : Outport  Port=2
  "gap " : Outport  Port=3  VectorParamsAs1DForOutWhenUnconnected=off
  unsafeFlag : Outport  Port=4  VectorParamsAs1DForOutWhenUnconnected=off
  wires:
  Mux2/1 -> errors/1
  velFilterReset/1 -> Integrator1/2
  Sum6/1 -> Compare To Constant/1
  Sum7/1 -> Sum6/1  "safe  gap"
  min h/1 -> Product/1
  Compare To Constant/1 -> unsafeFlag/1
  Sum2/1 -> Mux2/1  "eg"
  Bus Selector1/1 -> Sum/2  "<X>"
  Product/1 -> Sum7/2
  Sum3/1 -> Sum2/2  "desired  gap"
  Sum1/1 -> Sum/1  "x (front bumber)"
  Bus Selector2/2 -> Sum4/1, Multiply/1, Product/2  "<Xdot>"
  d0/1 -> Sum3/2
  vLen/1 -> Sum1/1
  min d0/1 -> Sum7/1
  Multiply/1 -> Sum3/1
  Sum/1 -> Sum2/1, "gap "/1, Sum6/2  "gap"
  Bus Selector2/1 -> Sum1/2  "<X>"
  h/1 -> Multiply/2, Multiply1/1
  Bus Selector1/2 -> Sum8/1  "<Xdot>"
  Sum4/1 -> Mux2/2, Sum10/1  "ev"
  Gain3/1 -> Saturation/1
  Saturation/1 -> Integrator1/1
  Integrator1/1 -> Sum4/2, Sum8/2
  Sum8/1 -> Gain3/1
  Bus Selector1/3 -> Sum9/2  "<xddot>"
  Bus Selector2/3 -> Sum9/1, Multiply1/2  "<xddot>"
  Multiply1/1 -> Sum10/2
  Sum10/1 -> Mux3/1  "egDot"
  Sum9/1 -> Mux3/2  "evDot"
  Mux3/1 -> errorsDot/1
  ego/1 -> Bus Selector2/1
  leader/1 -> Bus Selector1/1

== system full_maneuver_single_veh/Ld/Regular Vehicle Following/Define Desired Distance ==
  extraSpaceFlag : Inport
  Constant : Constant  Value=h
  Constant1 : Constant  Value=d0
  Constant2 : Constant  Value=hLC
  Constant3 : Constant  Value=d0LC
  Demux : Demux  Outputs=2
  Integrator : Integrator  InitialCondition=[h d0]
  Mux : Mux  Inputs=2
  Mux1 : Mux  Inputs=2
  Saturation1 : Saturate  UpperLimit=hFilterSaturation  LowerLimit=-hFilterSaturation
  Sum5 : Sum  Inputs=|+-
  Switch : Switch  Criteria=u2 > Threshold
  hFilterGain : Gain  Gain=hFilterGain
  h : Outport
  d0 : Outport  Port=2
  wires:
  Mux/1 -> Switch/3
  Constant/1 -> Mux/1
  hFilterGain/1 -> Saturation1/1
  Constant2/1 -> Mux1/1
  Sum5/1 -> hFilterGain/1
  Mux1/1 -> Switch/1
  Switch/1 -> Sum5/1
  Constant3/1 -> Mux1/2
  Constant1/1 -> Mux/2
  extraSpaceFlag/1 -> Switch/2
  Saturation1/1 -> Integrator/1
  Integrator/1 -> Demux/1, Sum5/2
  Demux/1 -> h/1
  Demux/2 -> d0/1

== system full_maneuver_single_veh/Ld/Regular Vehicle Following/Veh Following ==
  errors : Inport
  errorsDot : Inport  Port=2
  realInput : Inport  Port=3
  leaderChange : Inport  Port=4
  inRange : Inport  Port=5
  Demux : Demux  Outputs=2
  Demux1 : Demux  Outputs=2
  Gain : Gain  Gain=Ka
  Gain1 : Gain  Gain=Kdd
  Gain3 : Gain  Gain=10
  Integrator1 : Integrator  ExternalReset=rising  InitialConditionSource=external  InitialCondition=vx0
  Kd : Gain  Gain=Kd
  Kp : Gain  Gain=Kp
  Saturation : Saturate  UpperLimit=inf  LowerLimit=minAcceleration
  Saturation1 : Saturate  UpperLimit=maxGapError  LowerLimit=minGapError
  Scope : Scope  NumInputPorts=6
  Sum : Sum  Inputs=+-|
  Sum1 : Sum  Inputs=+++++
  Sum8 : Sum  Inputs=|+-
  Transport Delay : TransportDelay  DelayTime=0.1
  integralTerm : Subsystem
  u : Outport  VectorParamsAs1DForOutWhenUnconnected=off
  wires:
  Kp/1 -> Sum1/2, Scope/2
  Gain3/1 -> Saturation/1
  Sum8/1 -> Gain3/1
  Saturation/1 -> Integrator1/1
  Integrator1/1 -> u/1, Sum8/2
  errors/1 -> Demux/1
  Saturation1/1 -> integralTerm/1(eh), Kp/1
  Demux/2 -> Kd/1  "ev"
  Kd/1 -> Sum1/3, Scope/3
  Demux/1 -> Saturation1/1  "eg"
  leaderChange/1 -> integralTerm/3(leaderChange)
  inRange/1 -> Integrator1/2, integralTerm/Enable
  Transport Delay/1 -> Sum1/1, Scope/1
  realInput/1 -> Sum/2, Integrator1/3
  Sum/1 -> integralTerm/2(inputDiff)
  integralTerm/1(Out1) -> Transport Delay/1
  Gain1/1 -> Sum1/4, Scope/4
  Gain/1 -> Sum1/5, Scope/5
  Sum1/1 -> Sum8/1, Sum/1, Scope/6
  errorsDot/1 -> Demux1/1
  Demux1/1 -> Gain1/1  "egDot"
  Demux1/2 -> Gain/1  "evDot"

== system full_maneuver_single_veh/Ld/Regular Vehicle Following/Velocity Control ==
  ev : Inport
  ea : Inport  Port=2
  realInput : Inport  Port=3
  Abs : Abs
  Compare To Constant : simulink/Logic and Bit Operations/Compare To Constant  relop=<=  const=0.5  OutDataTypeStr=boolean
  Constant : Constant  Value=0.05
  Gain : Gain  Gain=velKd
  Scope : Scope  NumInputPorts=4
  Sum : Sum  Inputs=++|
  Sum1 : Sum  Inputs=|-+
  Sum3 : Sum  Inputs=+++
  Transport Delay : TransportDelay  DelayTime=0.1
  integral term : Subsystem
  velKp : Gain  Gain=velKp
  u : Outport  VectorParamsAs1DForOutWhenUnconnected=off
  wires:
  Sum/1 -> u/1
  Constant/1 -> Sum/1
  Gain/1 -> Sum3/3, Scope/3
  ea/1 -> Gain/1
  realInput/1 -> Sum1/1
  Sum3/1 -> Transport Delay/1, Scope/4, Sum/2
  velKp/1 -> Sum3/2, Scope/2
  ev/1 -> integral term/1(ev), velKp/1
  Sum1/1 -> Abs/1
  Abs/1 -> Compare To Constant/1
  integral term/1(Out1) -> Scope/1, Sum3/1
  Compare To Constant/1 -> integral term/Enable
  Transport Delay/1 -> Sum1/2

== system full_maneuver_single_veh/Ld/Regular Vehicle Following/Velocity Error ==
  ego : Inport
  velRef : Inport  Port=2
  inRange : Inport  Port=3
  Bus Selector : BusSelector  OutputSignals=Xdot,xddot
  Gain : Gain  Gain=-1
  Gain3 : Gain  Gain=velFilterGain
  Integrator1 : Integrator  ExternalReset=rising  InitialCondition=vx0
  Saturation : Saturate  UpperLimit=maxComfAccel  LowerLimit=minComfAccel
  Sum : Sum  Inputs=+-|
  Sum8 : Sum  Inputs=|+-
  ev : Outport
  ea : Outport  Port=2
  wires:
  inRange/1 -> Integrator1/2
  Gain/1 -> ea/1
  Sum/1 -> ev/1
  Bus Selector/2 -> Gain/1  "<xddot>"
  Bus Selector/1 -> Sum/2  "<Xdot>"
  ego/1 -> Bus Selector/1
  Integrator1/1 -> Sum8/2, Sum/1
  velRef/1 -> Sum8/1
  Saturation/1 -> Integrator1/1
  Gain3/1 -> Saturation/1
  Sum8/1 -> Gain3/1

== system full_maneuver_single_veh/Ld/Regular Vehicle Following/switch ==
  errors : Inport
  errorsDot : Inport  Port=2
  gap : Inport  Port=3
  h : Inport  Port=4
  d0 : Inport  Port=5
  vRef : Inport  Port=6
  Compare To Constant : simulink/Logic and Bit Operations/Compare To Constant  relop=<=  const=0  OutDataTypeStr=boolean
  Demux1 : Demux  Outputs=2
  Gain1 : Gain
  MATLAB Function : MATLAB Function  TreatAsAtomicUnit=on
  Scope : Scope  NumInputPorts=2
  Selector : Selector  InputPortWidth=2  IndexOptions=Index vector (dialog)  Indices=[2]  OutputSizes=1
  Sum2 : Sum  Inputs=+-
  inRange : Outport  VectorParamsAs1DForOutWhenUnconnected=off
  wires:
  d0/1 -> MATLAB Function/2(d0)
  vRef/1 -> MATLAB Function/3(vRef)
  h/1 -> Gain1/1
  errors/1 -> Selector/1
  gap/1 -> Scope/1, Sum2/1
  Sum2/1 -> Compare To Constant/1
  Selector/1 -> MATLAB Function/4(ev)
  Compare To Constant/1 -> inRange/1
  Gain1/1 -> MATLAB Function/1(h)
  MATLAB Function/1(maxGap) -> Scope/2, Sum2/2
  errorsDot/1 -> Demux1/1
  Demux1/1 -> MATLAB Function/5(ehDot)
  Demux1/2 -> MATLAB Function/6(ea)

== system full_maneuver_single_veh/Ld/findLeader/Subsystem ==
  ego : Inport
  all : Inport  Port=2
  Enable : EnablePort
  MATLAB Function : MATLAB Function  TreatAsAtomicUnit=on
  idx : Outport  InitialOutput=1  VectorParamsAs1DForOutWhenUnconnected=off
  wires:
  all/1 -> MATLAB Function/2(allVehicles)
  MATLAB Function/1(leaderIdx) -> idx/1
  ego/1 -> MATLAB Function/1(ego)

== system full_maneuver_single_veh/Ld/findLeader/farAwayVeh ==
  ego : Inport  OutDataTypeStr=Bus: vehStatesBus
  Bus Assignment : BusAssignment  AssignedSignals=X
  Bus Selector : BusSelector  OutputSignals=X
  Constant : Constant  Value=1000
  Sum : Sum  Inputs=|++
  Out1 : Outport  OutDataTypeStr=Bus: vehStatesBus  VectorParamsAs1DForOutWhenUnconnected=off
  wires:
  ego/1 -> Bus Assignment/1, Bus Selector/1
  Constant/1 -> Sum/2
  Bus Assignment/1 -> Out1/1
  Bus Selector/1 -> Sum/1  "<X>"
  Sum/1 -> Bus Assignment/2  "X"

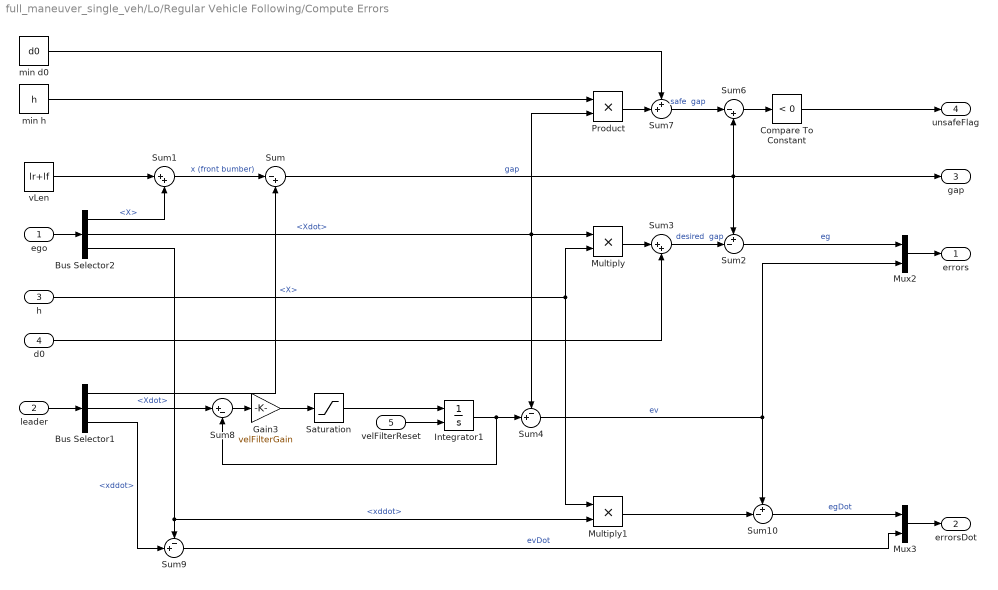
== system full_maneuver_single_veh/Lo/Regular Vehicle Following/Compute Errors ==
  ego : Inport
  leader : Inport  Port=2
  h : Inport  Port=3
  d0 : Inport  Port=4
  velFilterReset : Inport  Port=5
  Bus Selector1 : BusSelector  OutputSignals=X,Xdot,xddot
  Bus Selector2 : BusSelector  OutputSignals=X,Xdot,xddot
  Compare To Constant : simulink/Logic and Bit Operations/Compare To Constant  relop=<  const=0  OutDataTypeStr=boolean
  Gain3 : Gain  Gain=velFilterGain
  Integrator1 : Integrator  ExternalReset=rising  InitialCondition=vx0
  Multiply : Product
  Multiply1 : Product
  Mux2 : Mux  Inputs=2
  Mux3 : Mux  Inputs=2
  Product : Product
  Saturation : Saturate  UpperLimit=maxAcceleration  LowerLimit=minAcceleration
  Sum : Sum  Inputs=|-+
  Sum1 : Sum  Inputs=|++
  Sum10 : Sum  Inputs=+-|
  Sum2 : Sum  Inputs=+-|
  Sum3 : Sum  Inputs=|++
  Sum4 : Sum  Inputs=-+|
  Sum6 : Sum  Inputs=|-+
  Sum7 : Sum  Inputs=++|
  Sum8 : Sum  Inputs=|+-
  Sum9 : Sum  Inputs=-+|
  min d0 : Constant  Value=d0
  min h : Constant  Value=h
  vLen : Constant  Value=lr+lf
  errors : Outport  VectorParamsAs1DForOutWhenUnconnected=off
  errorsDot : Outport  Port=2
  "gap " : Outport  Port=3  VectorParamsAs1DForOutWhenUnconnected=off
  unsafeFlag : Outport  Port=4  VectorParamsAs1DForOutWhenUnconnected=off
  wires:
  leader/1 -> Bus Selector1/1
  ego/1 -> Bus Selector2/1
  Mux3/1 -> errorsDot/1
  Sum9/1 -> Mux3/2  "evDot"
  Sum10/1 -> Mux3/1  "egDot"
  Multiply1/1 -> Sum10/2
  Bus Selector2/3 -> Multiply1/2, Sum9/1  "<xddot>"
  Bus Selector1/3 -> Sum9/2  "<xddot>"
  Sum8/1 -> Gain3/1
  Integrator1/1 -> Sum8/2, Sum4/2
  Saturation/1 -> Integrator1/1
  Gain3/1 -> Saturation/1
  Sum4/1 -> Sum10/1, Mux2/2  "ev"
  Bus Selector1/2 -> Sum8/1  "<Xdot>"
  h/1 -> Multiply1/1, Multiply/2
  Bus Selector2/1 -> Sum1/2  "<X>"
  Sum/1 -> Sum6/2, "gap "/1, Sum2/1  "gap"
  Multiply/1 -> Sum3/1
  min d0/1 -> Sum7/1
  vLen/1 -> Sum1/1
  d0/1 -> Sum3/2
  Bus Selector2/2 -> Product/2, Multiply/1, Sum4/1  "<Xdot>"
  Sum1/1 -> Sum/1  "x (front bumber)"
  Sum3/1 -> Sum2/2  "desired  gap"
  Product/1 -> Sum7/2
  Bus Selector1/1 -> Sum/2  "<X>"
  Sum2/1 -> Mux2/1  "eg"
  Compare To Constant/1 -> unsafeFlag/1
  min h/1 -> Product/1
  Sum7/1 -> Sum6/1  "safe  gap"
  Sum6/1 -> Compare To Constant/1
  velFilterReset/1 -> Integrator1/2
  Mux2/1 -> errors/1

== system full_maneuver_single_veh/Lo/Regular Vehicle Following/Define Desired Distance ==
  extraSpaceFlag : Inport
  Constant : Constant  Value=h
  Constant1 : Constant  Value=d0
  Constant2 : Constant  Value=hLC
  Constant3 : Constant  Value=d0LC
  Demux : Demux  Outputs=2
  Integrator : Integrator  InitialCondition=[h d0]
  Mux : Mux  Inputs=2
  Mux1 : Mux  Inputs=2
  Saturation1 : Saturate  UpperLimit=hFilterSaturation  LowerLimit=-hFilterSaturation
  Sum5 : Sum  Inputs=|+-
  Switch : Switch  Criteria=u2 > Threshold
  hFilterGain : Gain  Gain=hFilterGain
  h : Outport
  d0 : Outport  Port=2
  wires:
  Demux/2 -> d0/1
  Demux/1 -> h/1
  Integrator/1 -> Sum5/2, Demux/1
  Saturation1/1 -> Integrator/1
  extraSpaceFlag/1 -> Switch/2
  Constant1/1 -> Mux/2
  Constant3/1 -> Mux1/2
  Switch/1 -> Sum5/1
  Mux1/1 -> Switch/1
  Sum5/1 -> hFilterGain/1
  Constant2/1 -> Mux1/1
  hFilterGain/1 -> Saturation1/1
  Constant/1 -> Mux/1
  Mux/1 -> Switch/3

== system full_maneuver_single_veh/Lo/Regular Vehicle Following/Veh Following ==
  errors : Inport
  errorsDot : Inport  Port=2
  realInput : Inport  Port=3
  leaderChange : Inport  Port=4
  inRange : Inport  Port=5
  Demux : Demux  Outputs=2
  Demux1 : Demux  Outputs=2
  Gain : Gain  Gain=Ka
  Gain1 : Gain  Gain=Kdd
  Gain3 : Gain  Gain=10
  Integrator1 : Integrator  ExternalReset=rising  InitialConditionSource=external  InitialCondition=vx0
  Kd : Gain  Gain=Kd
  Kp : Gain  Gain=Kp
  Saturation : Saturate  UpperLimit=inf  LowerLimit=minAcceleration
  Saturation1 : Saturate  UpperLimit=maxGapError  LowerLimit=minGapError
  Scope : Scope  NumInputPorts=6
  Sum : Sum  Inputs=+-|
  Sum1 : Sum  Inputs=+++++
  Sum8 : Sum  Inputs=|+-
  Transport Delay : TransportDelay  DelayTime=0.1
  integralTerm : Subsystem
  u : Outport  VectorParamsAs1DForOutWhenUnconnected=off
  wires:
  Demux1/2 -> Gain/1  "evDot"
  Demux1/1 -> Gain1/1  "egDot"
  errorsDot/1 -> Demux1/1
  Sum1/1 -> Scope/6, Sum/1, Sum8/1
  Gain/1 -> Scope/5, Sum1/5
  Gain1/1 -> Scope/4, Sum1/4
  integralTerm/1(Out1) -> Transport Delay/1
  Sum/1 -> integralTerm/2(inputDiff)
  realInput/1 -> Integrator1/3, Sum/2
  Transport Delay/1 -> Scope/1, Sum1/1
  inRange/1 -> integralTerm/Enable, Integrator1/2
  leaderChange/1 -> integralTerm/3(leaderChange)
  Demux/1 -> Saturation1/1  "eg"
  Kd/1 -> Scope/3, Sum1/3
  Demux/2 -> Kd/1  "ev"
  Saturation1/1 -> Kp/1, integralTerm/1(eh)
  errors/1 -> Demux/1
  Integrator1/1 -> Sum8/2, u/1
  Saturation/1 -> Integrator1/1
  Sum8/1 -> Gain3/1
  Gain3/1 -> Saturation/1
  Kp/1 -> Scope/2, Sum1/2

== system full_maneuver_single_veh/Lo/Regular Vehicle Following/Velocity Control ==
  ev : Inport
  ea : Inport  Port=2
  realInput : Inport  Port=3
  Abs : Abs
  Compare To Constant : simulink/Logic and Bit Operations/Compare To Constant  relop=<=  const=0.5  OutDataTypeStr=boolean
  Constant : Constant  Value=0.05
  Gain : Gain  Gain=velKd
  Scope : Scope  NumInputPorts=4
  Sum : Sum  Inputs=++|
  Sum1 : Sum  Inputs=|-+
  Sum3 : Sum  Inputs=+++
  Transport Delay : TransportDelay  DelayTime=0.1
  integral term : Subsystem
  velKp : Gain  Gain=velKp
  u : Outport  VectorParamsAs1DForOutWhenUnconnected=off
  wires:
  Transport Delay/1 -> Sum1/2
  Compare To Constant/1 -> integral term/Enable
  integral term/1(Out1) -> Sum3/1, Scope/1
  Abs/1 -> Compare To Constant/1
  Sum1/1 -> Abs/1
  ev/1 -> velKp/1, integral term/1(ev)
  velKp/1 -> Scope/2, Sum3/2
  Sum3/1 -> Sum/2, Scope/4, Transport Delay/1
  realInput/1 -> Sum1/1
  ea/1 -> Gain/1
  Gain/1 -> Scope/3, Sum3/3
  Constant/1 -> Sum/1
  Sum/1 -> u/1

== system full_maneuver_single_veh/Lo/Regular Vehicle Following/Velocity Error ==
  ego : Inport
  velRef : Inport  Port=2
  inRange : Inport  Port=3
  Bus Selector : BusSelector  OutputSignals=Xdot,xddot
  Gain : Gain  Gain=-1
  Gain3 : Gain  Gain=velFilterGain
  Integrator1 : Integrator  ExternalReset=rising  InitialCondition=vx0
  Saturation : Saturate  UpperLimit=maxComfAccel  LowerLimit=minComfAccel
  Sum : Sum  Inputs=+-|
  Sum8 : Sum  Inputs=|+-
  ev : Outport
  ea : Outport  Port=2
  wires:
  Sum8/1 -> Gain3/1
  Gain3/1 -> Saturation/1
  Saturation/1 -> Integrator1/1
  velRef/1 -> Sum8/1
  Integrator1/1 -> Sum/1, Sum8/2
  ego/1 -> Bus Selector/1
  Bus Selector/1 -> Sum/2  "<Xdot>"
  Bus Selector/2 -> Gain/1  "<xddot>"
  Sum/1 -> ev/1
  Gain/1 -> ea/1
  inRange/1 -> Integrator1/2
